simulink model "untitled1"  (R2023b)
settings: Solver=VariableStepAuto  StartTime=0.0  StopTime=10.0  RelTol=1e-3
settings Model: Creator=Rabin  LastModifiedBy=Rabin

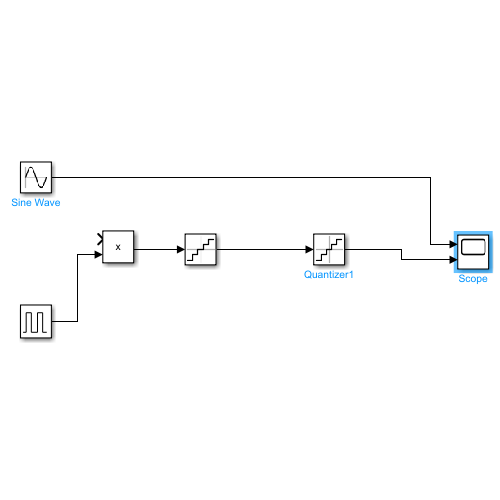
[thumbnail: Simulink's stored preview of the top-level diagram]
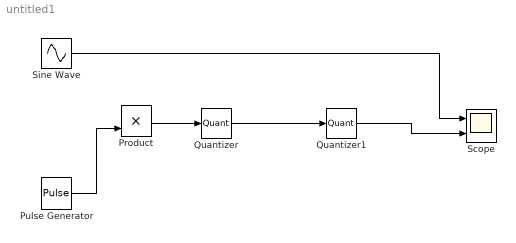
== system untitled1 ==
  Product : Product
  Pulse Generator : DiscretePulseGenerator  PulseType=Time based  Period=10  PulseWidth=5
  Quantizer : Quantizer
  Quantizer1 : Quantizer
  Scope : Scope  NumInputPorts=2
  Sine Wave : Sin  SampleTime=0
  wires:
  Pulse Generator/1 -> Product/2
  Product/1 -> Quantizer/1
  Quantizer/1 -> Quantizer1/1
  Quantizer1/1 -> Scope/2
  Sine Wave/1 -> Scope/1
